simulink model "simTest"  (R2018a)
settings: Solver=FixedStepAuto  StartTime=0  StopTime=180  FixedStep=0.005  RelTol=1e-3
model workspace: external: MAT-File (data not in the file)
undefined symbols (not defined in the file or in its folder): QINITIAL
libraries: libCarbo x1
settings Model: SnapshotBufferSize=1  SnapshotInterval=1  Creator=aordonez  LastModifiedBy=alejandro
settings SolverCC: AlgebraicLoopSolver=LineSearch
settings DataIOCC: SaveFormat=Array  ReturnWorkspaceOutputs=on
settings SFSimCC: SimUseLocalCustomCode=on
settings RTWCC: RTWUseLocalCustomCode=on
settings CodeAppCC: StateflowObjectComments=on

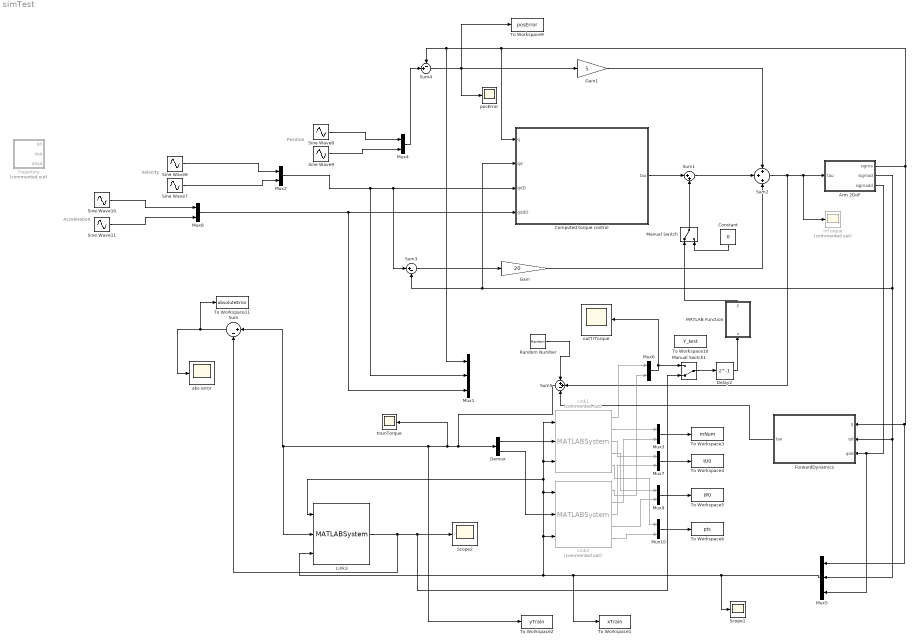
== system simTest ==
  note: Velocity
  note: Position
  note: Acceleration
  Arm 2DoF : Subsystem
  Computed torque control : MATLAB Function  TreatAsAtomicUnit=on
  Constant : Constant  Value=0
  Delay2 : Delay  DelayLength=1
  Demux : Demux  Outputs=2
  ForwardDynamics : MATLAB Function  TreatAsAtomicUnit=on
  Gain : Gain  Gain=20
  Gain1 : Gain  Gain=5
  InTorque : Scope  Commented=on
  Link1 : MATLABSystem  Commented=on  System=DLGP_IE  pts=50  N=10000  xSize=6  timeRate=0.005  divMethod=3  wo=100  loadHyp=off  fileName=name  sigN=1  sigF=1  lengthScale=1
      mask Type: DLGP_IE
      mask Display:
      | disp('DLGP1');
      | port_label('input',1,'xTrain');
      | port_label('input',2,'yTrain');
      | port_label('input',3,'xTest');
      | port_label('output',1,'yTest');
      | port_label('output',2,'mN');
      | port_label('output',3,'tU');
      | port_label('output',4,'tP');
      | port_label('output',5,'pts');
  Link2 : MATLABSystem  Commented=on  System=DLGP_IE  pts=50  N=10000  xSize=6  timeRate=0.005  divMethod=3  wo=100  loadHyp=off  fileName=name  sigN=1  sigF=1  lengthScale=1
      mask Type: DLGP_IE
      mask Display:
      | disp('DLGP1');
      | port_label('input',1,'xTrain');
      | port_label('input',2,'yTrain');
      | port_label('input',3,'xTest');
      | port_label('output',1,'yTest');
      | port_label('output',2,'mN');
      | port_label('output',3,'tU');
      | port_label('output',4,'tP');
      | port_label('output',5,'pts');
  Link3 : MATLABSystem  System=DLGP_IE_M  outs=2  pts=50  N=10000  xSize=6  timeRate=0.005  divMethod=3  wo=100  loadHyp=off  fileName=name  sigN=[1,1]  sigF=[1,1]  lengthScale=[1,1]
      mask Type: DLGP_IE_M
      mask Display:
      | disp('DLGP1');
      | port_label('input',1,'xTrain');
      | port_label('input',2,'yTrain');
      | port_label('input',3,'xTest');
      | port_label('output',1,'yTest');
  MATLAB Function : MATLAB Function  TreatAsAtomicUnit=on
  Manual Switch : ManualSwitch
  Manual Switch1 : ManualSwitch  CurrentSetting=0
  Mux1 : Mux  Inputs=3
  Mux{2..4,6..10} (8 alike) : Mux  Inputs=2
  Mux5 : Mux  Inputs=3
  Random Number : RandomNumber  SampleTime=0.005
  Scope1 : Scope
  Scope2 : Scope
  Sine Wave10 : Sin  Amplitude=-pi/6  Phase=pi/2  SampleTime=0
  Sine Wave11 : Sin  Amplitude=-pi/24  Frequency=0.5  Phase=pi/2  SampleTime=0
  Sine Wave6 : Sin  Amplitude=-pi/6  SampleTime=0
  Sine Wave7 : Sin  Amplitude=-pi/12  Frequency=0.5  SampleTime=0
  Sine Wave8 : Sin  Amplitude=pi/6  Phase=pi/2  SampleTime=0
  Sine Wave9 : Sin  Amplitude=pi/6  Frequency=0.5  Phase=pi/2  SampleTime=0
  Sum : Sum  Inputs=|+-
  Sum1 : Sum  Inputs=|++
  Sum2 : Sum  Inputs=+++
  Sum3 : Sum  Inputs=|+-
  Sum4 : Sum  Inputs=-+|
  Sum5 : Sum  Inputs=++-
  To Workspace1 : ToWorkspace  VariableName=xTrain  SampleTime=-1
      settings: Save2DSignal=2-D array (concatenate along first dimension)
  To Workspace10 : ToWorkspace  VariableName=Y_test  SampleTime=-1
      settings: Save2DSignal=2-D array (concatenate along first dimension)
  To Workspace11 : ToWorkspace  VariableName=absoluteError  SampleTime=-1
      settings: Save2DSignal=2-D array (concatenate along first dimension)
  To Workspace2 : ToWorkspace  VariableName=yTrain  SampleTime=-1
      settings: Save2DSignal=2-D array (concatenate along first dimension)
  To Workspace3 : ToWorkspace  VariableName=mNum  SampleTime=-1
      settings: Save2DSignal=2-D array (concatenate along first dimension)
  To Workspace4 : ToWorkspace  VariableName=tU0  SampleTime=-1
      settings: Save2DSignal=2-D array (concatenate along first dimension)
  To Workspace5 : ToWorkspace  VariableName=tP0  SampleTime=-1
      settings: Save2DSignal=2-D array (concatenate along first dimension)
  To Workspace6 : ToWorkspace  VariableName=pts  SampleTime=-1
      settings: Save2DSignal=2-D array (concatenate along first dimension)
  To Workspace9 : ToWorkspace  VariableName=posError  SampleTime=-1
      settings: Save2DSignal=2-D array (concatenate along first dimension)
  Trajectory : Subsystem  Commented=on
  abs error : Scope
  outTrTorque : Scope
  posError : Scope
  trainTorque : Scope
  wires:
  Sum4/1 -> posError/1, Gain1/1, To Workspace9/1
  Mux4/1 -> Sum4/2
  Arm 2DoF/1(sigma) -> Mux5/1, ForwardDynamics/1(q), Computed torque control/1(q), Mux1/1, Sum4/1
  Sum3/1 -> Gain/1
  Computed torque control/1(tau) -> Sum1/1
  Sum1/1 -> Sum2/2
  Sum2/1 -> Sum5/2, InTorque/1, Arm 2DoF/1(tau)
  Gain1/1 -> Sum2/1
  Gain/1 -> Sum2/3
  Arm 2DoF/2(sigmad) -> Computed torque control/2(qd), Sum3/2, Mux5/2, ForwardDynamics/2(qd)
  Demux/1 -> Link1/2
  Link1/1 -> Mux6/1
  Link2/1 -> Mux6/2
  Sine Wave6/1 -> Mux2/1
  Sine Wave7/1 -> Mux2/2
  Sine Wave10/1 -> Mux8/1
  Sine Wave11/1 -> Mux8/2
  Sine Wave8/1 -> Mux4/1
  Sine Wave9/1 -> Mux4/2
  Arm 2DoF/3(sigmadd) -> Mux5/3, ForwardDynamics/3(qdd)
  Sum/1 -> To Workspace11/1, abs error/1
  Demux/2 -> Link2/2
  Random Number/1 -> Sum5/1
  Mux2/1 -> Mux1/2, Sum3/1, Computed torque control/3(qdD)
  Mux8/1 -> Mux1/3, Computed torque control/4(qddD)
  Manual Switch/1 -> Sum1/2
  Constant/1 -> Manual Switch/2
  Mux6/1 -> Manual Switch1/1, outTrTorque/1
  Link1/2 -> Mux3/1
  Link2/2 -> Mux3/2
  Mux3/1 -> To Workspace3/1
  Link1/3 -> Mux7/1
  Link2/3 -> Mux7/2
  Link1/4 -> Mux9/1
  Link2/4 -> Mux9/2
  Link1/5 -> Mux10/1
  Link2/5 -> Mux10/2
  Mux10/1 -> To Workspace6/1
  Mux9/1 -> To Workspace5/1
  Mux7/1 -> To Workspace4/1
  MATLAB Function/1(y) -> Manual Switch/1
  Mux5/1 -> Scope1/1, Link2/1, Link3/1, Link1/3, Link1/1, Link2/3, Link3/3, To Workspace1/1
  Sum5/1 -> Demux/1, Link3/2, Sum/1, To Workspace2/1, trainTorque/1
  Delay2/1 -> MATLAB Function/1(u)
  ForwardDynamics/1(tau) -> Sum5/3
  Manual Switch1/1 -> Delay2/1
  Link3/1 -> Sum/2, Manual Switch1/2, Scope2/1

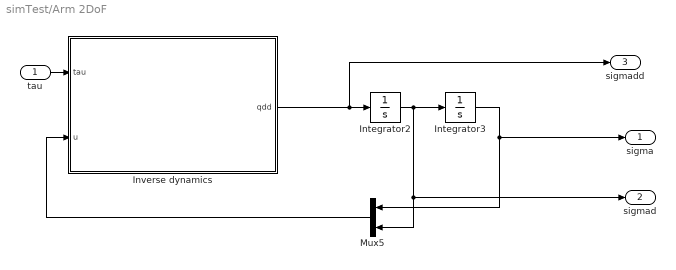
== system simTest/Arm 2DoF ==
  tau : Inport
  Integrator2 : Integrator  InitialCondition=[0;0]
  Integrator3 : Integrator  InitialCondition=[0;0]
  Inverse dynamics : MATLAB Function  TreatAsAtomicUnit=on
  Mux5 : Mux  Inputs=2
  sigma : Outport
  sigmad : Outport  Port=2
  sigmadd : Outport  Port=3
  wires:
  Integrator3/1 -> sigma/1, Mux5/1
  tau/1 -> Inverse dynamics/1(tau)
  Integrator2/1 -> sigmad/1, Mux5/2, Integrator3/1
  Mux5/1 -> Inverse dynamics/2(u)
  Inverse dynamics/1(qdd) -> Integrator2/1, sigmadd/1

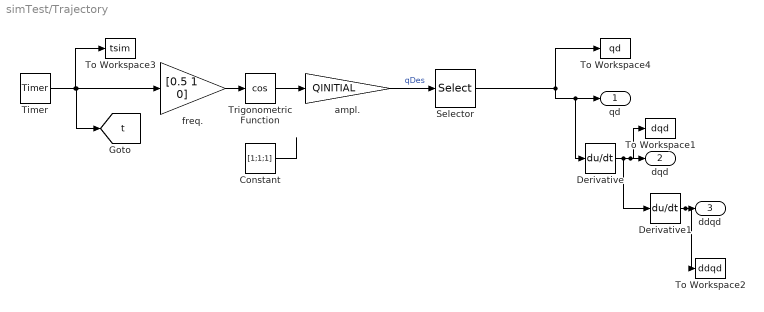
== system simTest/Trajectory ==
  Constant : Constant  Value=[1;1;1]
  Derivative : Derivative
  Derivative1 : Derivative
  Selector : Selector  InputPortWidth=3  IndexOptions=Index vector (dialog)  Indices=[1 2]  OutputSizes=1
  Timer : libCarbo/Timer
  To Workspace1 : ToWorkspace  VariableName=dqd  SampleTime=-1
  To Workspace2 : ToWorkspace  VariableName=ddqd  SampleTime=-1
  To Workspace3 : ToWorkspace  VariableName=tsim  SampleTime=-1
  To Workspace4 : ToWorkspace  VariableName=qd  SampleTime=-1
  Trigonometric Function : Trigonometry  Operator=cos
  ampl. : Gain  Gain=QINITIAL
  freq. : Gain  Gain=[0.5 1 0]
  qd : Outport
  dqd : Outport  Port=2
  ddqd : Outport  Port=3
  tag scope: t=global
  wires:
  Timer/1 -> freq./1, [t], To Workspace3/1
  freq./1 -> Trigonometric Function/1
  Trigonometric Function/1 -> ampl./1
  Derivative/1 -> Derivative1/1, To Workspace1/1, dqd/1
  Derivative1/1 -> ddqd/1, To Workspace2/1
  ampl./1 -> Selector/1  "qDes"
  Selector/1 -> Derivative/1, qd/1, To Workspace4/1
  Constant/1 -> ?

== matlab function simTest/ForwardDynamics ==
  data: q input; tau output; qd input; qdd input
function tau = CTcontrol(q,qd,qdd)
%{
inverse dynamics of a 2 DoF robotic arm

Inputs q: 2x1 vector. desired angular position
       qd: 2x1 vector. desired angular velocity
       qdd: 2x1 vector. desired angular acceleration

Output tau: 2x1 vector. Torques
%}
constant = 1.9;
Iz1 = constant;   %moment of inertia
Iz2 =constant;    
m1 = constant;    %mass
m2 = constant;
l1 = constant;    %length
l2 = constant;
r1 = l1;   %length to the center of mass
r2 = l2;
g = 9.81;  %gravity

a = Iz1 + Iz2 + m1*r1^2 + m2*( l1^2 + r2^2 );
b = m2*l1*r2;
d = Iz2 + m2*r2^2;

M = [ a + 2*b*cos( q(2) ),   d + b*cos( q(2) );
          d + b*cos( q(2) ),              d        ];

C = [ -b*sin( q(2) )*qd(2)     , -b*sin( q(2) )*( qd(1) + qd(2) );
       b*sin( q(2) )*qd(1)     ,               0                  ];

N = [ m1*g*r1*cos( q(1) ) + m2*g*( l1*cos( q(1) ) + r2*cos( q(1)+q(2) ) );
                    m2*g*r2*cos( q(1)+q(2) )                              ];
                
tau = M*(qdd) + C*(qd) +N;

== matlab function simTest/Computed torque control ==
  data: q input; tau output; qd input; qdD input; qddD input
function tau = CTcontrol(q,qd,qdD,qddD)
%{
inverse dynamics of a 2 DoF robotic arm

Inputs q: 2x1 vector. given angular position
       qd: 2x1 vector. given angular velocity
       qdD: 2x1 vector. desired angular velocity 
       qddD: 2x1 vector. desired angular acceleration

Output tau: 2x1 vector. Torques
%}
constant = 1.9;
Iz1 = constant;   %moment of inertia
Iz2 =constant;    
m1 = constant;    %mass
m2 = constant;
l1 = constant;    %length
l2 = constant;
r1 = l1;   %length to the center of mass
r2 = l2;
g = 9.81;  %gravity

a = Iz1 + Iz2 + m1*r1^2 + m2*( l1^2 + r2^2 );
b = m2*l1*r2;
d = Iz2 + m2*r2^2;

M = [ a + 2*b*cos( q(2) ),   d + b*cos( q(2) );
          d + b*cos( q(2) ),              d        ];

C = [ -b*sin( q(2) )*qd(2)     , -b*sin( q(2) )*( qd(1) + qd(2) );
       b*sin( q(2) )*qd(1)     ,               0                  ];

N = [ m1*g*r1*cos( q(1) ) + m2*g*( l1*cos( q(1) ) + r2*cos( q(1)+q(2) ) );
                    m2*g*r2*cos( q(1)+q(2) )                              ];
                
tau = M*(qddD) + C*(qdD) +N;

== matlab function simTest/MATLAB Function ==
  data: u input; y output
function y = slidingWindow(u)

persistent uold
WS = 30; 
Nu = 2; 
if isempty(uold)
    uold = zeros(Nu,WS);
end
uold(:,2:end) = uold(:,1:end-1);
uold(:,1) = u;
y = sum(uold,2)/WS;

== matlab function simTest/Arm 2DoF/Inverse dynamics ==
  data: tau input; u input; qdd output
function qdd = fcn(tau,u)
%{
inverse dynamics of a 2 DoF robotic arm
Inputs tau: 2x1 vector. Torques
       u: 4x1 vector [sigma1, sigma2, sigma1d, sigma2d]' position and speed
Output qdd: 2x1 vector with accelerations 
%}

Iz1 = 2;   %moment of inertia
Iz2 =2;    
m1 = 2;    %mass
m2 = 2;
l1 = 2;    %length
l2 = 2;
r1 = 2;   %length to the center of mass
r2 = 2;
g = 9.81;  %gravity

a = Iz1 + Iz2 + m1*r1^2 + m2*( l1^2 + r2^2 );
b = m2*l1*r2;
d = Iz2 + m2*r2^2;

M_inv = [ a + 2*b*cos( u(2) ),   d + b*cos( u(2) );
          d + b*cos( u(2) ),              d        ]^-1;

C = [ -b*sin( u(2) )*(2*u(3)*u(4) + u(4)^2); 
            b*sin( u(2) )*u(3)^2           ];
        

N = [ m1*g*r1*cos( u(1) ) + m2*g*( l1*cos( u(1) ) + r2*cos( u(1)+u(2) ) );
                    m2*g*r2*cos( u(1)+u(2) )                              ];

qdd = M_inv*( -C - N  + tau );
